simulink model "PLANTA_COMPLETA_CN2_MATLAB"  (R2024b)
settings: Solver=FixedStepAuto  StartTime=0.0  StopTime=inf  FixedStep=0.001  MaxStep=0.0005  RelTol=1e-4
InitFcn:
  | load('ml_breakpoints.mat')
  | load('l_breakpoints.mat')
  | load('at_breakpoints.mat')
  | load('Kp_table.mat')
  | load('Kd_table.mat')
undefined symbols (not defined in the file): A_hm, A_tm, at_breakpoints, at_max, b_ha, B_hm, b_ta, B_tm, bcx, bcy, bhd, bhEb, bhm, bt, btd, btm, btw, bwu, C_hm, C_tm, D_hm, D_tm, dl_h_ini, dx_l_ini, dx_t_ini, dx_td_ini, dxt_max, dy_l_ini, F01_a_t_max, F01_Ts1, F02_a_h_max, F02_Ts1, F03_a_h_max, F03_a_t_max, F03_dxt_max, F03_Ts1, Fhw_min, g, Hc, ih, it, Jhd_hEb, Jhm_hb, Jtd, Jtm_tb, K_hsa, K_hsia, K_tsa, K_tsia, Kcy, Kd_table, Kp_table, Ktw, kwu, l_breakpoints, l_h_ini, Lh0, Mc_max, ml_breakpoints, Ms ... (+21)
libraries: simulink x9, spsEdgeDetectorLib x5, simulink_extras x2, dspsigops x2, vrlib x1, dspstat3 x1
(part 1 of 3)
settings Model: Creator=ribei  LastModifiedBy=juani
settings SolverCC: ZeroCrossAlgorithm=Adaptive  AutoInsertRateTranBlk=on
settings DebuggingCC: IgnoredZcDiagnostic=none  UnderSpecifiedDimensionMsg=warning

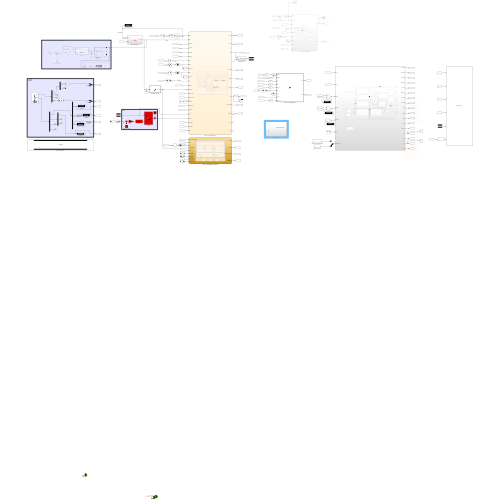
[thumbnail: Simulink's stored preview of the top-level diagram]
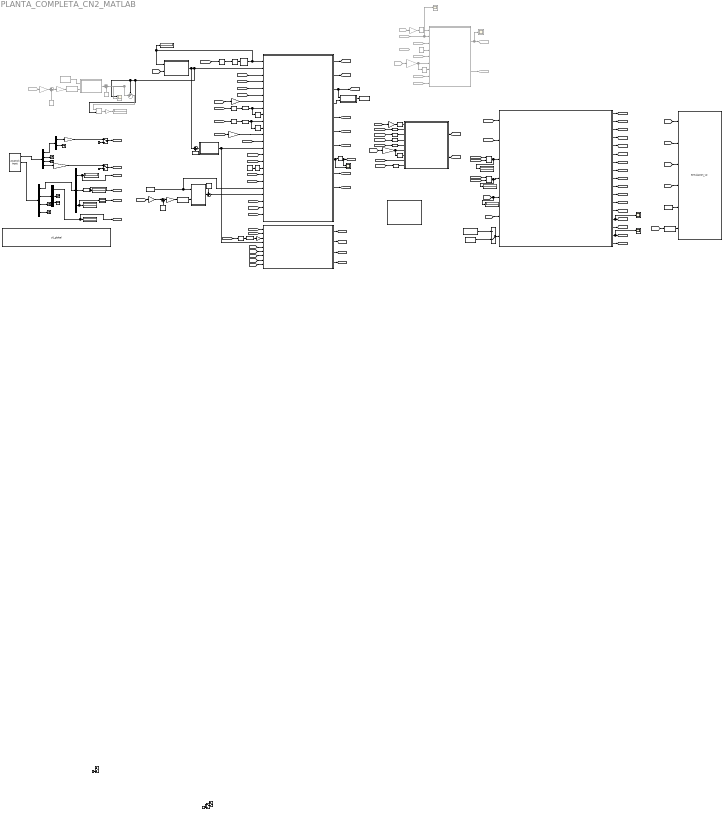
== system PLANTA_COMPLETA_CN2_MATLAB ==
  note: SOLO PARA PROBAR ESTIMADOR DE MASA
  note: HMI
  note: LIDAR
  AND : Logic  IconShape=distinctive  AllPortsSameDT=off  OutDataTypeStr=boolean
  AND1 : Logic  IconShape=distinctive  AllPortsSameDT=off  OutDataTypeStr=boolean
  Actualizar perfil : Subsystem
  Ajuste referencia : Constant  Value=30
  Ajuste referencia1 : Constant  Commented=on  Value=30
  Boton A : Display
  Boton B : Display
  Boton X : Display
  Boton Y : Display
  Calculo : MATLAB Function  Commented=on  TreatAsAtomicUnit=on
  Cast To Boolean : DataTypeConversion  OutDataTypeStr=boolean  SaturateOnIntegerOverflow=off  RndMeth=Floor
  Constant : Constant  Commented=on  Value=0
  Constant{1..2,18..19,28} (5 alike) : Constant  Value=0  SampleTime=T_s1
  Constant15 : Constant  Value=Yt0
  Constant3 : Constant  Commented=on  Value=Ms
  Constant4 : Constant
  Constant9 : Constant  Value=Ms
  Data Store Read1 : DataStoreRead  DataStoreName=y0_global  IndexOptions=Index vector (dialog)  Indices=1  OutputSizes=1
  Data Store Read2 : DataStoreRead  DataStoreName=y0_global  IndexOptions=Index vector (dialog)  Indices=1  OutputSizes=1
  Data Store Write : DataStoreWrite  DataStoreName=y0_global  IndexOptions=Index vector (dialog)  Indices=1  OutputSizes=1
  Data Type Conversion : DataTypeConversion  OutDataTypeStr=int32  RndMeth=Ceiling  SaturateOnIntegerOverflow=off
  Data Type Conversion1 : DataTypeConversion  Commented=on  OutDataTypeStr=int32  RndMeth=Ceiling  SaturateOnIntegerOverflow=off
  Delay{,3..6} (5 alike) : Delay  DelayLength=1  InputProcessing=Columns as channels (frame based)
  Delay1 : Delay  DelayLength=1  InputProcessing=Columns as channels (frame based)  SampleTime=T_s1
  Delay2 : Delay  DelayLength=1  InputProcessing=Columns as channels (frame based)  SampleTime=T_s1
  Demux : Demux
  Demux1 : Demux  Outputs=2
  Demux2 : Demux
  Demux3 : Demux  Outputs=3
  Demux4 : Demux  Outputs=3
  Derivative : Derivative  Commented=on
  Derivative1 : Derivative  Commented=on
  Derivative2 : Derivative
  Derivative3 : Derivative
  Discrete Derivative : simulink/Discrete/Discrete Derivative  gainval=1.0  ICPrevScaledInput=0.0  OutMin=[]  OutMax=[]  OutDataType=fixdt(1, 16)  OutScaling=2^-10  DoSatur=off
  Discrete Derivative1 : simulink/Discrete/Discrete Derivative  gainval=1.0  ICPrevScaledInput=0.0  OutMin=[]  OutMax=[]  OutDataType=fixdt(1, 16)  OutScaling=2^-10  DoSatur=off
  Discrete Derivative2 : simulink/Discrete/Discrete Derivative  gainval=1.0  ICPrevScaledInput=0.0  OutMin=[]  OutMax=[]  OutDataType=fixdt(1, 16)  OutScaling=2^-10  DoSatur=off
  Display{,2..4} (4 alike) : Display
  Display1 : Display  Commented=on
  Divide : Product  Commented=on  Inputs=*/
  Enclavamiento : Stateflow chart  TreatAsAtomicUnit=on
  Enclavamiento1 : Stateflow chart  TreatAsAtomicUnit=on
  From1 : From  Commented=on  GotoTag=tita_l
  From11 : From  Commented=on  GotoTag=dxt_ref
  From15 : From  Commented=on  GotoTag=Ml_estimada
  From2 : From  Commented=on  GotoTag=tita_tm
  From21 : From  Commented=on  GotoTag=bal_control
  From22 : From  Commented=on  GotoTag=ddxt_ref
  From3 : From  Commented=on  GotoTag=tita_hm
  From44 : From  Commented=on  GotoTag=dlh_ref
  From5 : From  Commented=on  GotoTag=tita_tm
  Gain : Gain  Gain=1/Wc
  Gain1 : Gain  Commented=on  Gain=rtd/it
  Gain10 : Gain  Gain=rtd/it
  Gain11 : Gain  Gain=-rhd/(ih*2)
  Gain2 : Gain  Commented=on  Gain=-rhd/(ih*2)
  Gain3 : Gain  Gain=rtd/it
  Gain4 : Gain  Gain=rtd/it
  Gain5 : Gain  Gain=-rhd/(ih*2)
  Gain6 : Gain  Commented=on  Gain=1/Wc
  Gain7 : Gain  Commented=on  Gain=rtd/it
  Gain8 : Gain  Gain=rhd/(-2*ih)
  Gain9 : Gain  Commented=on  Gain=100
  Goto10 : Goto  Commented=on  GotoTag=T_tm
  Goto11 : Goto  Commented=on  GotoTag=T_hm
  Joystick Input : vrlib/Joystick Input  joyid=1  adjustports=on  forcefeed=off
  Level-2 MATLAB S-Function : M-S-Function  FunctionName=Simulacion_v2  Parameters=2.438, 2.591, 1.500, 0.850, 0.750, 7.500, 2.100, 2.500, 'black', 'black', '#E99000', 5.000
  Manual Switch{1..4,11} (5 alike) : ManualSwitch
  Manual Switch5 : ManualSwitch  CurrentSetting=0
  Masa contenedor : Subsystem
  Memory1 : Memory  InheritSampleTime=on
  Moving Average : dspstat3/Moving Average  Method=Sliding window  ForgettingFactorPort=off  SpecifyWindowLength=on  WindowLength=40  OverlapLength=0  AllowArbitraryInputLength=off  ForgettingFactor=0.9  SimulateUsing=Interpreted execution
  Multiply : Gain  Gain=vt_max
  Multiply1 : Gain  Gain=vh_max_sc
  Nivel 0 - Seguridad o Proteccion : Stateflow chart  TreatAsAtomicUnit=on  SystemSampleTime=T_s0
      settings: PortSchema="{\"entries\":[{\"content\":{\"sides\":[{\"content\":{\"connectorIds\":[\"In6\",\"In9\",\"In8\",\"In7\",\"In1\",\"In2\",\"In3\",\"In5\",\"In4\"]},\"type\":\"ConnectorPlacement.EquallySpacedRectSide\",\"uuid\":\"92abb5b4-7f8d-4d16-9e1c-3f1528aec02e\"},{\"content\":{\"connectorIds\":[\"Out2\",\"Out1\",\"Out3\",\"Out4\"],\"side\":\"RIGHT\"},\"type\":\"ConnectorPlacement.EquallySpacedRectSide\",\"uuid\":\"fdfc4918-925b-4492-9924-9f3ed7c6f0ea\"},{\"content\":{\"side\":\"TOP\"},\"type\":\"ConnectorPlacement.EquallySpacedRectSide\",\"uuid\":\"6cd2c614-9727-439b-b51b-96ebe361e1e6\"},{\"content\":{\"side\":\"BOTTOM\"},\"type\":\"ConnectorPlacement.EquallySpacedRectSide\",\"uuid\":\"c327f02f-ffd6-4494-8eea-bb6a75c04a8c\"}]},\"type\":\"ConnectorPlacement.EquallySpacedConnector\",\"uuid\":\"17c891de-27fd-4863-a62e-79c0c94ffbc9\"}],\"packageUris\":[\"http://schema.mathworks.com/mf0/Connector/R2020b\"],\"version\":\"1.0\"}"
  Nivel 1 - Control Supervisor : Stateflow chart  TreatAsAtomicUnit=on  SystemSampleTime=T_s1
  Nivel 2 - Control Regulatorio : Subsystem  Commented=on
  Nivel 2: Control Regulatorio : MATLAB Function  TreatAsAtomicUnit=on  SystemSampleTime=T_s2
  Perfil de obstaculos : DataStoreMemory  DataStoreName=y0_global  WriteAfterWriteMsg=warning  InitialValue=y0  ShowAdditionalParam=off  OutDataTypeStr=double
  Scope : Scope
  Scope1 : Scope  Commented=on  NumInputPorts=2
  Scope2 : Scope  NumInputPorts=2
  Scope3 : Scope
  Scope4 : Scope  Commented=on
  Scope5 : Scope  Commented=on
  Slider Gain : simulink/Math Operations/Slider Gain  gain=27  low=-80  high=50
  Subsystem : Subsystem
  Subsystem1 : Subsystem
  Sum : Sum  Inputs=|++
  Sum1 : Sum  Inputs=|++
  Sum2 : Sum  Inputs=+-|
  Sum3 : Sum  Commented=on  Inputs=|++
  Sum4 : Sum  Commented=on  Inputs=|++
  Sum5 : Sum  Commented=on  Inputs=-|+||
  Tapped Delay : simulink/Discrete/Tapped Delay  vinit=0.0  samptime=T_s1  NumDelays=40  DelayOrder=Oldest  includeCurrent=off
  Terminator{,1..6} (7 alike) : Terminator
  Vector de masas : FromWorkspace  VariableName=Mc_Xvect
  Vector de masas sobrecarga : FromWorkspace  VariableName=Mc_Xvect_sobrecarga
  Vector de masas3 : FromWorkspace  Commented=on  VariableName=Mc_Xvect
  Velocidad max izaje : MATLAB Function  TreatAsAtomicUnit=on
  Zero-Order Hold : ZeroOrderHold  SampleTime=T_s1
  Zero-Order Hold1 : ZeroOrderHold  SampleTime=T_s1
  Zero-Order Hold2 : ZeroOrderHold  SampleTime=T_s1
  Zero-Order Hold3 : ZeroOrderHold  SampleTime=T_s0
  sensor : MATLAB Function  TreatAsAtomicUnit=on
  wires:
  AND/1 -> Display/1, Subsystem1/3(BRK_t)
  AND1/1 -> Display3/1, Subsystem1/4(BRK_h)
  Subsystem1/12(tita_tm) -> [tita_tm]
  Subsystem1/13(tita_hm) -> [tita_hm]
  Subsystem1/14(x_t) -> Scope/1, [x_t]
  Subsystem1/15(x_l) -> [x_l]
  Subsystem1/16(y_l) -> Scope3/1, [y_l]
  Data Store Read2/1 -> Level-2 MATLAB S-Function/5
  [tita_l] -> Level-2 MATLAB S-Function/4
  Gain2/1 -> Derivative1/1, Nivel 2 - Control Regulatorio/6(l_h)
  From3/1 -> Gain2/1
  From15/1 -> Nivel 2 - Control Regulatorio/3(m_l)
  Nivel 2 - Control Regulatorio/1(T_tm) -> Goto10/1, Scope4/1
  From2/1 -> Gain1/1  "signal"
  Gain1/1 -> Derivative/1
  Masa contenedor/1(Mc_X) -> Nivel 1 - Control Supervisor/2(Ml), Sum5/1, Scope1/1, Divide/2, Sum1/1  "signal"
  [FC_SUP] -> Nivel 1 - Control Supervisor/3(FC_SUP)  "signal"
  [FC_INF] -> Nivel 1 - Control Supervisor/4(FC_INF)  "signal"
  [FC_IZQ] -> Nivel 1 - Control Supervisor/5(FC_IZQ)  "signal"
  [FC_DER] -> Nivel 1 - Control Supervisor/6(FC_DER)  "signal"
  Gain3/1 -> Nivel 1 - Control Supervisor/7(xtd)  "signal"
  [tita_hm] -> Zero-Order Hold/1  "signal"
  [tita_tm] -> Zero-Order Hold1/1  "signal"
  Gain5/1 -> Nivel 1 - Control Supervisor/12(lh)  "signal"
  [falla_E] -> Nivel 1 - Control Supervisor/13(falla_E)
  Demux4/1 -> [Boton_A], Boton A/1  "signal"
  Demux4/2 -> Enclavamiento1/1(input)  "signal"
  Slider Gain/1 -> Nivel 1 - Control Supervisor/17(destino)  "signal"
  Nivel 1 - Control Supervisor/3(TLK) -> [TLK], Actualizar perfil/1(TLK)
  Nivel 1 - Control Supervisor/7(BRK_t) -> [BRK_t_N1]
  Nivel 1 - Control Supervisor/6(BRK_h) -> [BRK_h_N1]
  Nivel 1 - Control Supervisor/5(bal_control) -> [bal_control]
  Nivel 1 - Control Supervisor/4(c) -> Actualizar perfil/2(index)
  Nivel 2 - Control Regulatorio/2(T_hm) -> Goto11/1
  [T_tm] -> Subsystem1/1(T_tm)
  [T_hm] -> Subsystem1/2(T_hm)
  [BRK_hE] -> Display4/1, Subsystem1/5(BRK_hE)
  Subsystem1/11(tita_l) -> [tita_l]
  [x_t] -> Level-2 MATLAB S-Function/1
  [x_l] -> Level-2 MATLAB S-Function/2
  [y_l] -> Level-2 MATLAB S-Function/3
  Subsystem1/1(FC_IZQ) -> [FC_IZQ]
  Subsystem1/2(FCE_IZQ) -> [FCE_IZQ]
  Subsystem1/3(FC_DER) -> [FC_DER]
  Subsystem1/4(FCE_DER) -> [FCE_DER]
  Subsystem1/5(FC_INF) -> [FC_INF]
  Subsystem1/6(FCE_INF) -> [FCE_INF]
  Subsystem1/7(FC_SUP) -> [FC_SUP]
  Subsystem1/8(FCE_SUP) -> [FCE_SUP]
  Subsystem1/9(Fhw) -> [Fhw]
  Subsystem1/10(S_TLK) -> [S_TLK]
  [tita_tm] -> Gain3/1  "signal"
  Discrete Derivative1/1 -> Nivel 1 - Control Supervisor/10(wtm), Delay1/1
  [tita_hm] -> Gain5/1
  Actualizar perfil/1(y0_actualizado) -> Data Store Write/1
  Data Type Conversion/1 -> sensor/2(index)
  Constant15/1 -> Sum2/1
  sensor/1(distancia) -> Sum2/2
  Ajuste referencia/1 -> Sum/2
  Gain4/1 -> Sum/1  "xtd"
  Sum/1 -> Gain/1
  Gain/1 -> Data Type Conversion/1
  [tita_tm] -> Gain4/1  "signal"
  Subsystem1/17(Ftw) -> [Ftw]
  Nivel 1 - Control Supervisor/1(dxt_ref) -> [dxt_ref]  "dxt_ref"
  Nivel 1 - Control Supervisor/2(dlh_ref) -> [dlh_ref]  "dlh_ref"
  Derivative/1 -> Nivel 2 - Control Regulatorio/1(dx_td)  "dx_td"
  Derivative1/1 -> Nivel 2 - Control Regulatorio/7(dl_h)
  From11/1 -> Scope5/1, Nivel 2 - Control Regulatorio/2(dx_tref)  "dxt_ref"
  From44/1 -> Nivel 2 - Control Regulatorio/5(dl_href)
  Demux/1 -> Demux1/1
  Demux/3 -> Terminator1/1
  Demux1/2 -> Terminator2/1
  Demux/2 -> Terminator/1
  Joystick Input/1 -> Demux/1
  Constant28/1 -> Manual Switch11/2
  ? -> Manual Switch11/1
  Constant1/1 -> Manual Switch1/2
  ? -> Manual Switch1/1
  Constant2/1 -> Manual Switch2/2
  Constant18/1 -> Manual Switch3/2
  Demux1/1 -> Multiply/1  "Carro"
  Constant19/1 -> Manual Switch4/2
  Demux/4 -> Multiply1/1  "Izaje"
  Demux3/1 -> [Boton_Y], Boton Y/1
  Demux3/2 -> Terminator5/1
  Demux4/3 -> Enclavamiento/1(input), Boton X/1
  Demux2/2 -> Demux3/1
  Demux2/4 -> Terminator4/1
  Demux3/3 -> Terminator6/1
  Joystick Input/2 -> Demux2/1
  Demux2/3 -> Terminator3/1
  Demux2/1 -> Demux4/1
  Sum1/1 -> Velocidad max izaje/1(M_l)
  Constant9/1 -> Sum1/2
  [TLK] -> Masa contenedor/2(TLK)
  Velocidad max izaje/1(dxt_max) -> Nivel 1 - Control Supervisor/14(dlh_max), Nivel 0 - Seguridad o Proteccion/7(v_max_izaje)  "signal"
  Multiply1/1 -> Manual Switch4/1
  Discrete Derivative/1 -> Nivel 1 - Control Supervisor/8(whm), Delay2/1
  Delay1/1 -> Nivel 1 - Control Supervisor/11(wtm_ant)
  Zero-Order Hold/1 -> Discrete Derivative/1
  Zero-Order Hold1/1 -> Discrete Derivative1/1
  Sum2/1 -> Nivel 1 - Control Supervisor/21(yc0_xt)
  Data Store Read1/1 -> sensor/1(y0_array), Nivel 1 - Control Supervisor/20(Y_c0)
  [T_tm] -> Nivel 1 - Control Supervisor/22(Ttm_disp)
  [T_hm] -> Nivel 1 - Control Supervisor/23(Thm_disp)
  [Fhw] -> Zero-Order Hold2/1  "signal"
  Moving Average/1 -> Display2/1, Masa contenedor/1(Fwh), Nivel 1 - Control Supervisor/1(Fhw)  "señal filtrada"
  Tapped Delay/1 -> Moving Average/1
  Zero-Order Hold2/1 -> Tapped Delay/1  "señal cruda"
  Vector de masas3/1 -> Calculo/1(masas_array)
  Ajuste referencia1/1 -> Sum3/2
  Sum3/1 -> Gain6/1
  Data Type Conversion1/1 -> Calculo/2(index)
  Gain6/1 -> Data Type Conversion1/1
  From5/1 -> Gain7/1  "signal"
  Gain7/1 -> Sum3/1  "signal"
  Calculo/1(Mc_X) -> Sum4/1
  [TLK] -> Cast To Boolean/1
  Sum4/1 -> Sum5/2, Scope1/2  "Masa real"
  Constant3/1 -> Sum4/2
  Sum5/1 -> Divide/1
  Gain9/1 -> Display1/1
  Divide/1 -> Gain9/1
  Delay2/1 -> Nivel 1 - Control Supervisor/9(whm_ant)
  From1/1 -> Nivel 2 - Control Regulatorio/8(theta)
  Nivel 1 - Control Supervisor/9(Ml_estimada) -> [Ml_estimada]
  Constant/1 -> Nivel 2 - Control Regulatorio/4(BC)
  From22/1 -> Nivel 2 - Control Regulatorio/9(ddx_t_ref)
  Nivel 1 - Control Supervisor/10(ddxt_ref) -> [ddxt_ref]  "ddxt_ref"
  Multiply/1 -> Manual Switch3/1
  [tita_l] -> Nivel 1 - Control Supervisor/24(tita_l)
  Constant4/1 -> Slider Gain/1
  Manual Switch5/1 -> Subsystem1/7(masas_array)
  Vector de masas/1 -> Manual Switch5/2
  Vector de masas sobrecarga/1 -> Manual Switch5/1
  [FCE_IZQ] -> Nivel 0 - Seguridad o Proteccion/3(FCE_IZQ)
  [FCE_DER] -> Nivel 0 - Seguridad o Proteccion/2(FCE_DER)
  [FCE_SUP] -> Nivel 0 - Seguridad o Proteccion/5(FCE_SUP)
  [FCE_INF] -> Nivel 0 - Seguridad o Proteccion/4(FCE_INF)
  Nivel 0 - Seguridad o Proteccion/2(BRK_t) -> [BRK_t_N0]
  Nivel 0 - Seguridad o Proteccion/1(BRK_h) -> [BRK_h_N0]
  Nivel 0 - Seguridad o Proteccion/3(EmergenciaNivel) -> [falla_E]
  [Boton_B] -> Nivel 1 - Control Supervisor/18(balanceo_on)
  [Boton_X] -> Nivel 1 - Control Supervisor/19(TLK_act)
  Enclavamiento/1(output) -> [Boton_X]  "X"
  [Boton_A] -> Nivel 0 - Seguridad o Proteccion/6(PulsadorEmergecia)
  [Boton_Y] -> Nivel 0 - Seguridad o Proteccion/9(OK)
  Manual Switch4/1 -> [dlh_ref_man]
  Manual Switch3/1 -> [dxt_ref_man]
  [dlh_ref_man] -> Nivel 1 - Control Supervisor/15(dlh_ref_man)
  [dxt_ref_man] -> Nivel 1 - Control Supervisor/16(dxt_ref_man)
  [tita_hm] -> Zero-Order Hold3/1  "signal"
  Zero-Order Hold3/1 -> Discrete Derivative2/1
  Discrete Derivative2/1 -> Gain8/1
  Gain8/1 -> Nivel 0 - Seguridad o Proteccion/8(dlh)
  [alive] -> Nivel 0 - Seguridad o Proteccion/1(alive)
  Nivel 0 - Seguridad o Proteccion/4(BRK_hE) -> [BRK_hE]
  [BRK_t_N0] -> AND/1
  [BRK_t_N1] -> AND/2
  [BRK_h_N0] -> AND1/1
  [BRK_h_N1] -> AND1/2
  Memory1/1 -> Scope2/1, [alive]
  Nivel 1 - Control Supervisor/8(alive) -> Scope2/2, Memory1/1
  [dxt_ref] -> Delay/1  "dxt_ref"
  Gain10/1 -> Derivative2/1
  [tita_tm] -> Gain10/1  "signal"
  Derivative2/1 -> Nivel 2: Control Regulatorio/1(dx_td)  "dx_td"
  Nivel 2: Control Regulatorio/1(T_tm) -> [T_tm]
  [TLK] -> Subsystem1/6(TLK)
  Cast To Boolean/1 -> Level-2 MATLAB S-Function/6
  Delay/1 -> Nivel 2: Control Regulatorio/2(dx_tref)
  Nivel 2: Control Regulatorio/2(T_hm) -> [T_hm]
  [dlh_ref] -> Delay3/1
  [tita_hm] -> Gain11/1
  Gain11/1 -> Nivel 2: Control Regulatorio/6(l_h), Derivative3/1
  Derivative3/1 -> Nivel 2: Control Regulatorio/7(dl_h)
  Delay3/1 -> Nivel 2: Control Regulatorio/5(dlh_ref)
  [bal_control] -> Delay6/1
  [Ml_estimada] -> Delay5/1
  [tita_l] -> Nivel 2: Control Regulatorio/8(theta)
  [ddxt_ref] -> Delay4/1
  Delay4/1 -> Nivel 2: Control Regulatorio/9(ddx_t_ref)
  Delay5/1 -> Nivel 2: Control Regulatorio/3(m_l)
  Delay6/1 -> Nivel 2: Control Regulatorio/4(BC)
  Enclavamiento1/1(output) -> [Boton_B], Boton B/1  "B"

== system PLANTA_COMPLETA_CN2_MATLAB/Actualizar perfil ==
  TLK : Inport
  index : Inport  Port=2
  Data Store Read3 : DataStoreRead  DataStoreName=y0_global  IndexOptions=Index vector (dialog)  Indices=1  OutputSizes=1
  Edge Detector1 : spsEdgeDetectorLib/Edge Detector  model=Either  ic=0  Ts=-1
      settings: LibrarySourceBlock=sps_lib/Control/Edge Detector
  Enabled Subsystem : Subsystem  TreatAsAtomicUnit=on
  Switch : Switch  Criteria=u2 > Threshold  SaturateOnIntegerOverflow=off  InputSameDT=off
  Unit Delay : UnitDelay  SampleTime=-1  HasFrameUpgradeWarning=on
  y0_actualizado : Outport
  wires:
  Unit Delay/1 -> Edge Detector1/1
  TLK/1 -> Unit Delay/1
  Edge Detector1/1 -> Switch/2, Enabled Subsystem/Enable
  Enabled Subsystem/1(y0_actualizado) -> Switch/1
  index/1 -> Enabled Subsystem/1(index)
  Switch/1 -> y0_actualizado/1
  Data Store Read3/1 -> Switch/3

== system PLANTA_COMPLETA_CN2_MATLAB/Masa contenedor ==
  Fwh : Inport
  TLK : Inport  Port=2
  Edge Detector : spsEdgeDetectorLib/Edge Detector  model=Falling  ic=0  Ts=-1
      settings: LibrarySourceBlock=sps_lib/Control/Edge Detector
  Edge Detector1 : spsEdgeDetectorLib/Edge Detector  model=Rising  ic=0  Ts=-1
      settings: LibrarySourceBlock=sps_lib/Control/Edge Detector
  Gain8 : Gain  Gain=2/g
  Product : Product
  S-R Flip-Flop : simulink_extras/Flip Flops/S-R Flip-Flop  initial_condition=0
  Unit Delay : UnitDelay  SampleTime=-1  HasFrameUpgradeWarning=on
  Mc_X : Outport
  wires:
  TLK/1 -> Unit Delay/1
  Edge Detector/1 -> S-R Flip-Flop/2
  Edge Detector1/1 -> S-R Flip-Flop/1
  S-R Flip-Flop/1 -> Product/2
  Product/1 -> Mc_X/1
  Unit Delay/1 -> Edge Detector1/1, Edge Detector/1
  Fwh/1 -> Gain8/1  "m estimada"
  Gain8/1 -> Product/1  "m estimada"

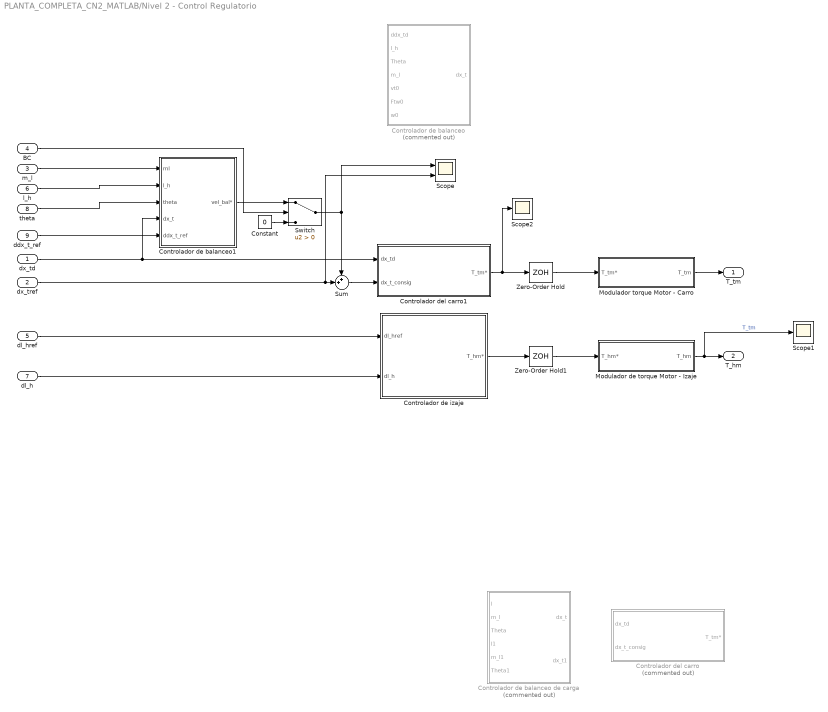
== system PLANTA_COMPLETA_CN2_MATLAB/Nivel 2 - Control Regulatorio ==
  dx_td : Inport
  dx_tref : Inport  Port=2
  m_l : Inport  Port=3
  BC : Inport  Port=4
  dl_href : Inport  Port=5
  l_h : Inport  Port=6
  dl_h : Inport  Port=7
  theta : Inport  Port=8
  ddx_t_ref : Inport  Port=9
  Constant : Constant  Value=0
  Controlador de balanceo : Subsystem  Commented=on
  Controlador de balanceo de carga : Subsystem  Commented=on
  Controlador de balanceo1 : Subsystem
  Controlador de izaje : Subsystem
  Controlador del carro : Subsystem  Commented=on
  Controlador del carro1 : Subsystem
  Modulador de torque Motor - Izaje : Subsystem
  Modulador torque Motor - Carro : Subsystem
  Scope : Scope  NumInputPorts=2
  Scope1 : Scope
  Scope2 : Scope
  Sum : Sum  Inputs=++|
  Switch : Switch  Criteria=u2 > Threshold  SaturateOnIntegerOverflow=off  InputSameDT=off
  Zero-Order Hold : ZeroOrderHold  SampleTime=T_s2
  Zero-Order Hold1 : ZeroOrderHold  SampleTime=T_s2
  T_tm : Outport
  T_hm : Outport  Port=2
  wires:
  dl_href/1 -> Controlador de izaje/1(dl_href)
  Zero-Order Hold1/1 -> Modulador de torque Motor - Izaje/1(T_hm*)
  dl_h/1 -> Controlador de izaje/2(dl_h)
  Controlador de izaje/1(T_hm*) -> Zero-Order Hold1/1
  Modulador de torque Motor - Izaje/1(T_hm) -> Scope1/1, T_hm/1  "T_tm"
  Zero-Order Hold/1 -> Modulador torque Motor - Carro/1(T_tm*)
  Modulador torque Motor - Carro/1(T_tm) -> T_tm/1
  l_h/1 -> Controlador de balanceo1/2(l_h)
  dx_td/1 -> Controlador del carro1/1(dx_td), Controlador de balanceo1/4(dx_t)
  Constant/1 -> Switch/3
  m_l/1 -> Controlador de balanceo1/1(ml)
  BC/1 -> Switch/2
  Controlador del carro1/1(T_tm*) -> Scope2/1, Zero-Order Hold/1
  Controlador de balanceo1/1(vel_bal*) -> Switch/1
  theta/1 -> Controlador de balanceo1/3(theta)
  dx_tref/1 -> Scope/2, Sum/2
  Sum/1 -> Controlador del carro1/2(dx_t_consig)
  Switch/1 -> Scope/1, Sum/1
  ddx_t_ref/1 -> Controlador de balanceo1/5(ddx_t_ref)

== system PLANTA_COMPLETA_CN2_MATLAB/Subsystem ==
  note: HMI DASHBOARD
  Lamp : CustomWebBlock  LabelPosition=Hide  ShowInitialText=on  Configuration="{\"components\":[{\"name\":\"BackgroundImageComponent\",\"settings\":{\"image\":{\"size\":[150,150],\"src\":\"data:image\\/svg+xml;base64,PHN2ZyB4bWxucz0iaHR0cDovL3d3dy53My5vcmcvMjAwMC9zdmciIHhtbG5zOnhsaW5rPSJodHRwOi8vd3d3LnczLm9yZy8xOTk5L3hsaW5rIiB2aWV3Qm94PSIwIDAgNTAwIDUwMCI+PGRlZnM+PHN0eWxlPi5he2ZpbGw6dXJsKCNhKTt9LmJ7ZmlsbDp1cmwoI2IpO30uY3tmaWxsOnVybCgjYyk7fTwvc3R5bGU+PHJhZGlhbEdyYWRpZW50IGlkPSJhIiBjeD0iMjgzLjg0IiBjeT0iLTQ2Ni4zNyIgcj0iMzc1Ljc1IiBncmFkaWVudFRyYW5zZm9ybT0ibWF0cml4KDEuMzksIDAsIDAsIC0xLjM5LCAtMTUzLjU2LCAtNjQ0LjA4KSIg ...(+2088 chars)\",\"srcOrientation\":\"Right\"},\"position\":[0,0,1,1],\"scaleMode\":\"0\"}},{\"name\":\"LampStateComponent\",\"settings\":{\"position\":[0,0,1,1],\"states\":[{\"icon\":{\"customSrc\":\"data:image\\/svg+xml;base64,PHN2ZyBpZD0iTGF5ZXJfMSIgZGF0YS1uYW1lPSJMYXllciAxIiB4bWxucz0iaHR0cDovL3d3dy53My5vcmcvMjAwMC9zdmciIHZpZXdCb3g9IjAgMCA0MTEgNDU4Ij48ZGVmcz48c3R5bGU+LmNscy0xe2ZpbGw6I2ZkZjhjMTt9LmNscy0ye2ZpbGw6I2ZlZTEwMDt9LmNscy0ze2ZpbGw6IzIzMWYyMDt9LmNscy00e2ZpbGw6I2EwOWY5Zjt9LmNscy00LC5jbHMtNSwuY2xzLTZ7c3Ryb2tlOiMyMzFmMjA7c3Ryb2tlLW1pdGVybGltaXQ6MTA7fS5jbHMtNXtmaWxsOiNmZmY7fS5jbHMtNntmaWxsOm5vbmU7fTwvc3R5bGU+PC9kZWZz ...(+5168 chars)\",\"id\":-1,\"srcOrientation\":\"Right\",\"type\":\"custom\"},\"iconScale\":0.8,\"metadata\":{},\"overlayType\":\"intersect\",\"shape\":{\"color\":[0.725,0,0],\"opacity\":1,\"position\":[0.1,0.1,0.8,0.8],\"type\":\"ellipse\"},\"value\":[]},{\"icon\":{\"customSrc\":\"data:image\\/svg+xml;base64,PHN2ZyBpZD0iTGF5ZXJfMSIgZGF0YS1uYW1lPSJMYXllciAxIiB4bWxucz0iaHR0cDovL3d3dy53My5vcmcvMjAwMC9zdmciIHZpZXdCb3g9IjAgMCA0MTEgNDU4Ij48ZGVmcz48c3R5bGU+LmNscy0xe2ZpbGw6I2ZkZjhjMTt9LmNscy0ye2ZpbGw6I2ZlZTEwMDt9LmNscy0ze2ZpbGw6IzIzMWYyMDt9LmNscy00e2ZpbGw6I2EwOWY5Zjt9LmNscy00LC5jbHMtNSwuY2xzLTZ7c3Ryb2tlOiMyMzFmMjA7c3Ryb2tlLW1pdGVybGltaXQ6MTA7fS5jbHMtNXtmaWxsOiNmZmY7fS5jbHMtNntmaWxsOm5vbmU7fTwvc3R5bGU+PC9kZWZz ...(+5168 chars)\",\"id\":-1,\"srcOrientation\":\"Right\",\"type\":\"custom\"},\"iconScale\":0.8,\"metadata\":{\"useDefaults\":{\"customIcon\":true,\"icon\":true,\"overlayType\":true,\"shape\":true,\"sizeAndPosition\":true}},\"overlayType\":\"intersect\",\"shape\":{\"color\":[0,0,0],\"opacity\":1,\"position\":[0.1,0.1,0.8,0.8],\"type\":\"ellipse\"},\"value\":\"0\"},{\"icon\":{\"customSrc\":\"data:image\\/svg+xml;base64,PHN2ZyBpZD0iTGF5ZXJfMSIgZGF0YS1uYW1lPSJMYXllciAxIiB4bWxucz0iaHR0cDovL3d3dy53My5vcmcvMjAwMC9zdmciIHZpZXdCb3g9IjAgMCA0MTEgNDU4Ij48ZGVmcz48c3R5bGU+LmNscy0xe2ZpbGw6I2ZkZjhjMTt9LmNscy0ye2ZpbGw6I2ZlZTEwMDt9LmNscy0ze2ZpbGw6IzIzMWYyMDt9LmNscy00e2ZpbGw6I2EwOWY5Zjt9LmNscy00LC5jbHMtNSwuY2xzLTZ7c3Ryb2tlOiMyMzFmMjA7c3Ryb2tlLW1pdGVybGltaXQ6MTA7fS5jbHMtNXtmaWxsOiNmZmY7fS5jbHMtNntmaWxsOm5vbmU7fTwvc3R5bGU+PC9kZWZz ...(+5168 chars)\",\"id\":-1,\"srcOrientation\":\"Right\",\"type\":\"custom\"},\"iconScale\":0.8,\"metadata\":{\"useDefaults\":{\"customIcon\":true,\"icon\":true,\"overlayType\":true,\"shape\":true,\"sizeAndPosition\":true}},\"overlayType\":\"intersect\",\"shape\":{\"color\":[0.39215686274509803,0.8313725490196079,0.07450980392156863],\"opacity\":1,\"position\":[0.1,0.1,0.8,0.8],\"type\":\"ellipse\"},\"value\":\"1\"}],\"valueType\":\"discrete\"}},{\"name\":\"ForegroundImageComponent\",\"settings\":{\"image\":{\"size\":[150,150],\"src\":\"data:image\\/svg+xml;base64,PHN2ZyB4bWxucz0iaHR0cDovL3d3dy53My5vcmcvMjAwMC9zdmciIHhtbG5zOnhsaW5rPSJodHRwOi8vd3d3LnczLm9yZy8xOTk5L3hsaW5rIiB2aWV3Qm94PSIwIDAgNTAwIDUwMCI+PGRlZnM+PHN0eWxlPi5he2ZpbGw6dXJsKCNhKTt9PC9zdHlsZT48bGluZWFyR3JhZGllbnQgaWQ9ImEiIHgxPSIxNzMuMDUiIHkxPSItNjI3Ljc4IiB4Mj0iMTczLjA1IiB5Mj0iLTUyMi40MyIgZ3JhZGllbnRUcmFuc2Zvcm09Im1hdHJpeCgxLjI5LCAwLCAwLCAtMS4zMywgMjcuMTMsIC02MjguMzEpIiBncmFkaWVudFVuaXRzPSJ1c2VyU3BhY2VPblVzZSI+PHN0b3Agb2Zmc2V0PSIwIiBzdG9wLWNvbG9yPSIjZmZmIiBzdG9wLW9wYWNpdHk9IjAuMjUiLz48c3RvcCBvZmZzZXQ9IjEiIHN0b3AtY29sb3I9IiNmZmYiIHN0b3Atb3BhY2l0eT0iMCIvPjwvbGluZWFyR3JhZGllbnQ+PC9kZWZzPjxwYXRoIGNsYXNzPSJhIiBkPSJNNDI5LjMsMTkwLjY2QzQwMi40NSwxMTQuNTEsMzMyLjY3LDYwLjE3LDI1MC44NSw2MC4xN2MtODMuNDMsMC0xNTQuMjgsNTYuNDItMTc5Ljk1LDEzNSwxNS4zNCwzOSw4OC4xMSw3LDE3Ny4wNyw3QzM0MCwyMDIuMDgsNDE3LjI2LDIzNi40Niw0MjkuMywxOTAuNjZaIi8+PC9zdmc+\",\"srcOrientation\":\"Right\"},\"isForeground\":1,\"position\":[0,0,1,1],\"scaleMode\":\"0\"}}],\"settings\":{\"BindingType\":\"signal\",\"aspectRatio\":1.032258064516129,\"backgroundColor\":[0,0,0],\"backgroundOffset\":0.14,\"backgroundOpacity\":1,\"blockOrientation\":\"Right\",\"fixedAspectRatio\":\"on\",\"showBackgroundColor\":false,\"value\":0,\"version\":\"R2023a\"},\"type\":\"Lamp\"}"  StateValueType=Discrete  Icon=Custom

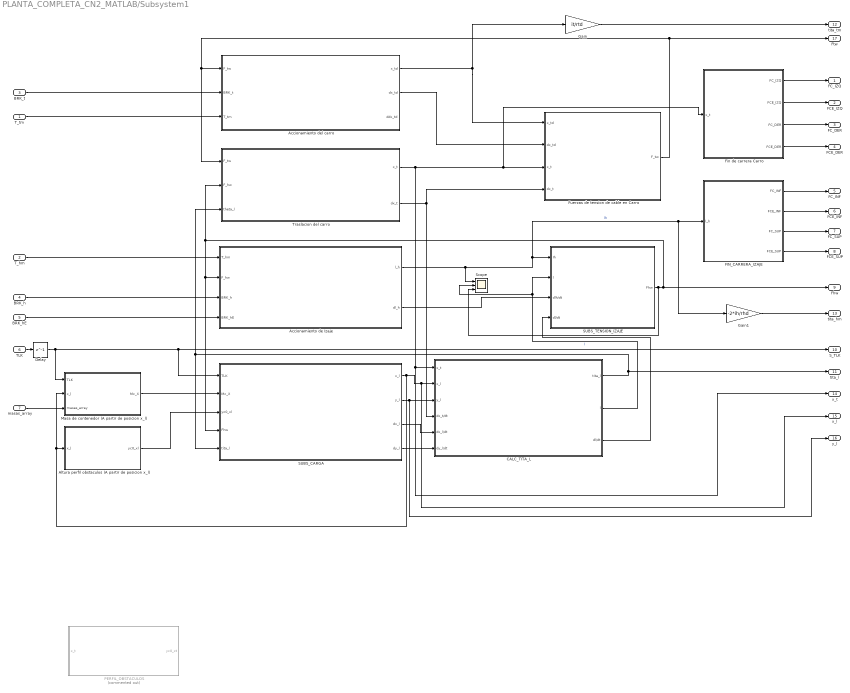
== system PLANTA_COMPLETA_CN2_MATLAB/Subsystem1 ==
  T_tm : Inport
  T_hm : Inport  Port=2
  BRK_t : Inport  Port=3
  BRK_h : Inport  Port=4
  BRK_hE : Inport  Port=5
  TLK : Inport  Port=6
  masas_array : Inport  Port=7
  Accionamiento de Izaje : Subsystem
  Accionamiento del carro : Subsystem
  Altura perfil obstaculos (A partir de posicion x_l) : Subsystem
  CALC_TITA_L : Subsystem
  Delay : Delay  DelayLength=1  InputProcessing=Columns as channels (frame based)  SampleTime=T_s1
  FIN_CARRERA_IZAJE : Subsystem
  Fin de carrera Carro : Subsystem
  Fuerzas de tension de cable en Carro : Subsystem
  Gain : Gain  Gain=it/rtd
  Gain1 : Gain  Gain=-2*ih/rhd
  Masa de contenedor (A partir de posicion x_l) : Subsystem
  PERFIL_OBSTACULOS : Subsystem  Commented=on
  SUBS_CARGA : Subsystem
  SUBS_TENSION_IZAJE : Subsystem
  Scope : Scope  NumInputPorts=3
  Traslacion del carro : Subsystem
  FC_IZQ : Outport
  FCE_IZQ : Outport  Port=2
  FC_DER : Outport  Port=3
  FCE_DER : Outport  Port=4
  FC_INF : Outport  Port=5
  FCE_INF : Outport  Port=6
  FC_SUP : Outport  Port=7
  FCE_SUP : Outport  Port=8
  Fhw : Outport  Port=9
  S_TLK : Outport  Port=10
  tita_l : Outport  Port=11
  tita_tm : Outport  Port=12
  tita_hm : Outport  Port=13
  x_t : Outport  Port=14
  x_l : Outport  Port=15
  y_l : Outport  Port=16
  Ftw : Outport  Port=17
  wires:
  Gain/1 -> tita_tm/1
  Traslacion del carro/2(dx_t) -> CALC_TITA_L/4(dx_t/dt), Fuerzas de tension de cable en Carro/4(dx_t)
  SUBS_TENSION_IZAJE/1(Fhw) -> Scope/3, Fhw/1, Traslacion del carro/2(F_hw), Accionamiento de Izaje/2(F_hw), SUBS_CARGA/4(Fhw)
  CALC_TITA_L/3(dl/dt) -> SUBS_TENSION_IZAJE/4(dl/dt)
  BRK_h/1 -> Accionamiento de Izaje/3(BRK_h)
  TLK/1 -> Delay/1
  BRK_t/1 -> Accionamiento del carro/2(BRK_t)
  Accionamiento del carro/1(x_td) -> Fuerzas de tension de cable en Carro/1(x_td), Gain/1
  BRK_hE/1 -> Accionamiento de Izaje/4(BRK_hE)
  Accionamiento del carro/2(dx_td) -> Fuerzas de tension de cable en Carro/2(dx_td)
  FIN_CARRERA_IZAJE/3(FC_SUP) -> FC_SUP/1
  Fin de carrera Carro/4(FCE_DER) -> FCE_DER/1
  SUBS_CARGA/4(dy_l) -> CALC_TITA_L/6(dy_l/dt)
  CALC_TITA_L/2(l) -> SUBS_TENSION_IZAJE/2(l), Scope/2  "l"
  Fuerzas de tension de cable en Carro/1(F_tw) -> Ftw/1, Accionamiento del carro/1(F_tw), Traslacion del carro/1(F_tw)
  SUBS_CARGA/3(dx_l) -> CALC_TITA_L/5(dx_l/dt)
  Altura perfil obstaculos (A partir de posicion x_l)/1(yc0_xl) -> SUBS_CARGA/3(yc0_xl)
  Accionamiento de Izaje/1(l_h) -> SUBS_TENSION_IZAJE/1(Ih), FIN_CARRERA_IZAJE/1(l_h), Gain1/1, Scope/1  "lh"
  Accionamiento de Izaje/2(dl_h) -> SUBS_TENSION_IZAJE/3(dlh/dt)
  T_tm/1 -> Accionamiento del carro/3(T_tm)
  Fin de carrera Carro/2(FCE_IZQ) -> FCE_IZQ/1
  T_hm/1 -> Accionamiento de Izaje/1(T_hm)
  FIN_CARRERA_IZAJE/1(FC_INF) -> FC_INF/1
  Gain1/1 -> tita_hm/1
  FIN_CARRERA_IZAJE/2(FCE_INF) -> FCE_INF/1
  Fin de carrera Carro/1(FC_IZQ) -> FC_IZQ/1
  FIN_CARRERA_IZAJE/4(FCE_SUP) -> FCE_SUP/1
  Fin de carrera Carro/3(FC_DER) -> FC_DER/1
  SUBS_CARGA/1(x_l) -> Masa de contenedor (A partir de posicion x_l)/2(x_l), Altura perfil obstaculos (A partir de posicion x_l)/1(x_l), x_l/1, CALC_TITA_L/2(x_l)
  CALC_TITA_L/1(tita_l) -> tita_l/1, Traslacion del carro/3(theta_l), SUBS_CARGA/5(tita_l)
  Traslacion del carro/1(x_t) -> CALC_TITA_L/1(x_t), x_t/1, Fin de carrera Carro/1(x_t), Fuerzas de tension de cable en Carro/3(x_t)
  SUBS_CARGA/2(y_l) -> y_l/1, CALC_TITA_L/3(y_l)
  Masa de contenedor (A partir de posicion x_l)/1(Mc_X) -> SUBS_CARGA/2(Mc_X)
  Delay/1 -> Masa de contenedor (A partir de posicion x_l)/1(TLK), S_TLK/1, SUBS_CARGA/1(TLK)
  masas_array/1 -> Masa de contenedor (A partir de posicion x_l)/3(masas_array)

== system PLANTA_COMPLETA_CN2_MATLAB/Actualizar perfil/Enabled Subsystem ==
  index : Inport
  Enable : EnablePort
  Actualiza perfil : MATLAB Function  TreatAsAtomicUnit=on
  Constant16 : Constant  Value=Hc
  Data Store Read3 : DataStoreRead  DataStoreName=y0_global  IndexOptions=Index vector (dialog)  Indices=1  OutputSizes=1
  y0_actualizado : Outport
  wires:
  Data Store Read3/1 -> Actualiza perfil/2(y0)
  Constant16/1 -> Actualiza perfil/3(Hc)
  index/1 -> Actualiza perfil/1(index)
  Actualiza perfil/1(y0_actualizado) -> y0_actualizado/1

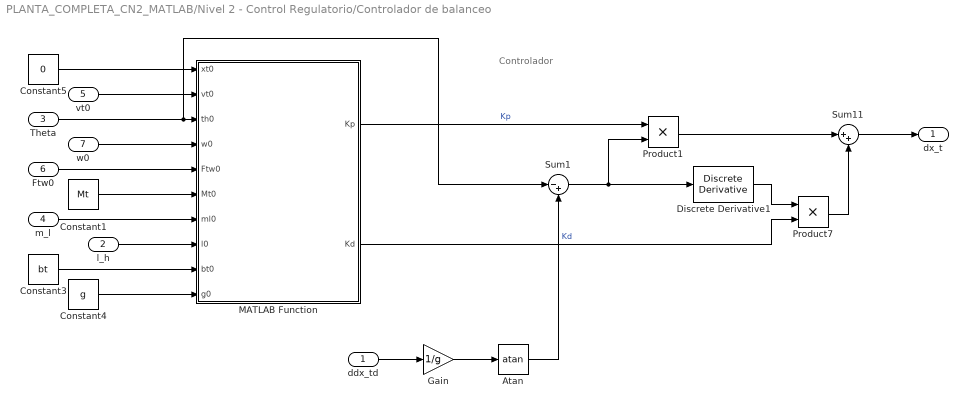
== system PLANTA_COMPLETA_CN2_MATLAB/Nivel 2 - Control Regulatorio/Controlador de balanceo ==
  note: Controlador
  ddx_td : Inport
  l_h : Inport  Port=2
  Theta : Inport  Port=3
  m_l : Inport  Port=4
  vt0 : Inport  Port=5
  Ftw0 : Inport  Port=6
  w0 : Inport  Port=7
  Atan : Trigonometry  Operator=atan
  Constant1 : Constant  Value=Mt
  Constant3 : Constant  Value=bt
  Constant4 : Constant  Value=g
  Constant5 : Constant  Value=0
  Discrete Derivative1 : simulink/Discrete/Discrete Derivative  gainval=1.0  ICPrevScaledInput=0.0  OutMin=[]  OutMax=[]  OutDataType=fixdt(1, 16)  OutScaling=2^-10  DoSatur=off
  Gain : Gain  Gain=1/g
  MATLAB Function : MATLAB Function  TreatAsAtomicUnit=on
  Product1 : Product
  Product7 : Product
  Sum1 : Sum  Inputs=|-+
  Sum11 : Sum  Inputs=|++
  dx_t : Outport
  wires:
  Discrete Derivative1/1 -> Product7/1
  Sum11/1 -> dx_t/1
  MATLAB Function/2(Kd) -> Product7/2  "Kd"
  Product7/1 -> Sum11/2
  Constant1/1 -> MATLAB Function/6(Mt0)
  m_l/1 -> MATLAB Function/7(ml0)
  Constant3/1 -> MATLAB Function/9(bt0)
  Constant4/1 -> MATLAB Function/10(g0)
  Constant5/1 -> MATLAB Function/1(xt0)
  vt0/1 -> MATLAB Function/2(vt0)
  w0/1 -> MATLAB Function/4(w0)
  ddx_td/1 -> Gain/1
  Gain/1 -> Atan/1
  l_h/1 -> MATLAB Function/8(l0)
  Atan/1 -> Sum1/2
  MATLAB Function/1(Kp) -> Product1/1  "Kp"
  Sum1/1 -> Discrete Derivative1/1, Product1/2
  Ftw0/1 -> MATLAB Function/5(Ftw0)
  Theta/1 -> Sum1/1, MATLAB Function/3(th0)
  Product1/1 -> Sum11/1
